simulink model "general_charger_2_precharge"  (R2013a)
settings: Solver=ode23  StartTime=0  StopTime=1.5  RelTol=1e-3
PreLoadFcn:
  | Ts =5e-6;
values from neighbouring files (symbols this model uses):
  ac_volt = 169    [charger_init.m]    (also in charger_init_simpl.m)
  acdc_on_time = 0.2    [charger_init.m]    (also in charger_init_simpl.m = 0)
  Cdc = 2e-3    (= 0.002)    [charger_init.m]    (also in charger_init_simpl.m)
  dcAd = dcinvexp*(eye(dcnstates) + (Ts/2)*dcAc)    [charger_init.m]    (also in charger_init_simpl.m)
  dcBd = dcinvexp*dcBc    [charger_init.m]    (also in charger_init_simpl.m)
  dcCd = dcCc*dcinvexp*Ts    [charger_init.m]    (also in charger_init_simpl.m)
  dcDd = dcCc*dcinvexp*dcBc*(Ts/2) + dcDc    [charger_init.m]    (also in charger_init_simpl.m)
  ESRCd = 70e-3    (= 0.07)    [charger_init.m]    (also in charger_init_simpl.m)
  ESRLdcdc = 0.1    [charger_init.m]    (also in charger_init_simpl.m)
  ESRLin = 0.2    [charger_init.m]    (also in charger_init_simpl.m = 0.1)
  Ldcdc = 1.3e-3    (= 0.0013)    [charger_init.m]    (also in charger_init_simpl.m = 0.0014)
  Lin = 1.5e-3    (= 0.0015)    [charger_init.m]    (also in charger_init_simpl.m = 0.001)
  P = 1.92e3    (= 1920)    [charger_init.m]    (also in charger_init_simpl.m)
  pre_charge_off = 0.2    [charger_init.m]
  pre_charge_r = 10    [charger_init.m]    (also in charger_init_simpl.m = 6)
  pre_charge_ramp = (dc_volt - Vdcmin)/(acdc_ramp_end_time - acdc_on_time)    (= 336.666666667)    [charger_init.m]    (also in charger_init_simpl.m = (dc_volt - Vdcmin)/(acdc_ramp_end_time - acdc_on_time))
  Q = 0    [charger_init.m]    (also in charger_init_simpl.m)
  Rbatt = 0.20    (= 0.2)    [charger_init.m]    (also in charger_init_simpl.m = 0.1)
  switch_Ts = 5e-5    (= 5e-05)    [charger_init.m]    (also in charger_init_simpl.m)
  sys_Ts = 5e-6    (= 5e-06)    [charger_init.m]    (also in charger_init_simpl.m)
  Vdcmin = ac_volt + 10    (= 179)    [charger_init.m]    (also in charger_init_simpl.m)
  voc = 105    [charger_init.m]    (also in charger_init_simpl.m)
undefined symbols (not defined in the file or in its folder): cpi
undefined symbols (not defined in the file): active_power_on, Ad, Bd, Cd, dc_volt, dcdc_cc_ref, dcdc_cv_ref, dcdc_iki, dcdc_ikp, dcdc_on, dcdc_vki, dcdc_vkp, Dd, dq_id_ki, dq_id_kp, dq_iq_ki, dq_iq_kp, dq_vdc_ki, dq_vdc_kp, dqQ_ki, dqQ_kp, P_ki, P_kp, pi_iac_ki, pi_iac_kp, pi_vdc_ki, pi_vdc_kp, piQ_ki, piQ_kp, pr_iac_kp, pr_pr_ki, pr_pr_kp, pr_vdc_ki, pr_vdc_kp, reactive_power_on
libraries: simulink_extras x165, powerlib x64, simulink x35, powerlib_meascontrol x11
(part 7 of 7)

== system general_charger_2_precharge/control_stage/AC//DC Control/DQ Controller/AB-DQ Transform/PLL/AB->DQ/Vd Discretization Error Correction/RMS4/PI3 ==
  in : Inport
  Add1 : Sum
  Add2 : Sum
  Ki : Gain  Gain=ki
  Kp : Gain  Gain=kp
  Tappe : simulink/Discrete/Tapped Delay  vinit=0.0  samptime=Ts_pi  NumDelays=1  DelayOrder=Oldest  includeCurrent=off
  Ts : Gain  Gain=Ts_pi
  integral saturation : Saturate  UpperLimit=int_sat_up  LowerLimit=int_sat_low  SampleTime=Ts_pi
  pi controller saturation : Saturate  UpperLimit=pi_sat_up  LowerLimit=pi_sat_low  SampleTime=Ts_pi
  out : Outport
  wires:
  Ts/1 -> Ki/1
  in/1 -> Kp/1, Ts/1  "vdc_error"
  Add1/1 -> integral saturation/1  "vdc_int_pi"
  Kp/1 -> Add2/2  "vdc_kp_pi"
  pi controller saturation/1 -> out/1
  Tappe/1 -> Add1/1
  Add2/1 -> pi controller saturation/1  "vdc_pi"
  Ki/1 -> Add1/2
  integral saturation/1 -> Add2/1, Tappe/1

== system general_charger_2_precharge/control_stage/AC//DC Control/DQ Controller/AB-DQ Transform/PLL/AB->DQ/Vq Discretization Error Correction/RMS4/PI3 ==
  in : Inport
  Add1 : Sum
  Add2 : Sum
  Ki : Gain  Gain=ki
  Kp : Gain  Gain=kp
  Tappe : simulink/Discrete/Tapped Delay  vinit=0.0  samptime=Ts_pi  NumDelays=1  DelayOrder=Oldest  includeCurrent=off
  Ts : Gain  Gain=Ts_pi
  integral saturation : Saturate  UpperLimit=int_sat_up  LowerLimit=int_sat_low  SampleTime=Ts_pi
  pi controller saturation : Saturate  UpperLimit=pi_sat_up  LowerLimit=pi_sat_low  SampleTime=Ts_pi
  out : Outport
  wires:
  Ts/1 -> Ki/1
  in/1 -> Kp/1, Ts/1  "vdc_error"
  Add1/1 -> integral saturation/1  "vdc_int_pi"
  Kp/1 -> Add2/2  "vdc_kp_pi"
  pi controller saturation/1 -> out/1
  Tappe/1 -> Add1/1
  Add2/1 -> pi controller saturation/1  "vdc_pi"
  Ki/1 -> Add1/2
  integral saturation/1 -> Add2/1, Tappe/1

== system general_charger_2_precharge/control_stage/AC//DC Control/PR Controller/PR Controller/PLL/AB->DQ/Vd Discretization Error Correction/RMS4/PI3 ==
  in : Inport
  Add1 : Sum
  Add2 : Sum
  Ki : Gain  Gain=ki
  Kp : Gain  Gain=kp
  Tappe : simulink/Discrete/Tapped Delay  vinit=0.0  samptime=Ts_pi  NumDelays=1  DelayOrder=Oldest  includeCurrent=off
  Ts : Gain  Gain=Ts_pi
  integral saturation : Saturate  UpperLimit=int_sat_up  LowerLimit=int_sat_low  SampleTime=Ts_pi
  pi controller saturation : Saturate  UpperLimit=pi_sat_up  LowerLimit=pi_sat_low  SampleTime=Ts_pi
  out : Outport
  wires:
  Ts/1 -> Ki/1
  in/1 -> Kp/1, Ts/1  "vdc_error"
  Add1/1 -> integral saturation/1  "vdc_int_pi"
  Kp/1 -> Add2/2  "vdc_kp_pi"
  pi controller saturation/1 -> out/1
  Tappe/1 -> Add1/1
  Add2/1 -> pi controller saturation/1  "vdc_pi"
  Ki/1 -> Add1/2
  integral saturation/1 -> Add2/1, Tappe/1

== system general_charger_2_precharge/control_stage/AC//DC Control/PR Controller/PR Controller/PLL/AB->DQ/Vq Discretization Error Correction/RMS4/PI3 ==
  in : Inport
  Add1 : Sum
  Add2 : Sum
  Ki : Gain  Gain=ki
  Kp : Gain  Gain=kp
  Tappe : simulink/Discrete/Tapped Delay  vinit=0.0  samptime=Ts_pi  NumDelays=1  DelayOrder=Oldest  includeCurrent=off
  Ts : Gain  Gain=Ts_pi
  integral saturation : Saturate  UpperLimit=int_sat_up  LowerLimit=int_sat_low  SampleTime=Ts_pi
  pi controller saturation : Saturate  UpperLimit=pi_sat_up  LowerLimit=pi_sat_low  SampleTime=Ts_pi
  out : Outport
  wires:
  Ts/1 -> Ki/1
  in/1 -> Kp/1, Ts/1  "vdc_error"
  Add1/1 -> integral saturation/1  "vdc_int_pi"
  Kp/1 -> Add2/2  "vdc_kp_pi"
  pi controller saturation/1 -> out/1
  Tappe/1 -> Add1/1
  Add2/1 -> pi controller saturation/1  "vdc_pi"
  Ki/1 -> Add1/2
  integral saturation/1 -> Add2/1, Tappe/1
